simulink model "OmniServerSim_v2021b"  (R2021b)
settings: Solver=FixedStepAuto  StartTime=0.0  StopTime=inf  FixedStep=0.002  MaxStep=1e-2  RelTol=1e-3
model workspace (MATLAB code in the model file):
  | % function MacroDef()
  | 
  | % //Omni端数据的state定义
  | % #define OMNI_SEND_STATE_ERROR -100
  | global OMNI_SEND_STATE_ERROR
  | OMNI_SEND_STATE_ERROR = (-100);
  | % #define OMNI_SEND_STATE_EMPTY 0
  | global OMNI_SEND_STATE_EMPTY
  | OMNI_SEND_STATE_EMPTY = (0);
  | % #define OMNI_SEND_STATE_HEARTBEAT 10
  | global OMNI_SEND_STATE_HEARTBEAT
  | OMNI_SEND_STATE_HEARTBEAT = (10);
  | % #define OMNI_SEND_STATE_SYN 20
  | global OMNI_SEND_STATE_SYN
  | OMNI_SEND_STATE_SYN = (20);
  | % #define OMNI_SEND_STATE_ONLY_NOTE 30
  | global OMNI_SEND_STATE_ONLY_NOTE
  | OMNI_SEND_STATE_ONLY_NOTE = (30);
  | % #define OMNI_SEND_STATE_CURRENT_CORE 100
  | global OMNI_SEND_STATE_CURRENT_CORE
  | OMNI_SEND_STATE_CURRENT_CORE = (100);
  | % #define OMNI_SEND_STATE_LAST_CORE 101
  | global OMNI_SEND_STATE_LAST_CORE
  | OMNI_SEND_STATE_LAST_CORE = (101);
  | % #define OMNI_SEND_STATE_CURRENT_POSE 200
  | global OMNI_SEND_STATE_CURRENT_POSE
  | OMNI_SEND_STATE_CURRENT_POSE = (200);
  | % #define OMNI_SEND_STATE_LAST_POSE 201
  | global OMNI_SEND_STATE_LAST_POSE
  | OMNI_SEND_STATE_LAST_POSE = (201);
  | % #define OMNI_SEND_STATE_CURRENT_FORCE 300
  | global OMNI_SEND_STATE_CURRENT_FORCE
  | OMNI_SEND_STATE_CURRENT_FORCE = (300);
  | % #define OMNI_SEND_STATE_LAST_FORCE 301
  | global OMNI_SEND_STATE_LAST_FORCE
  | OMNI_SEND_STATE_LAST_FORCE = (301);
  | % #define OMNI_RCV_STATE_EMPTY 1000
  | global OMNI_RCV_STATE_EMPTY
  | OMNI_RCV_STATE_EMPTY = (1000);
  | % #define OMNI_RCV_STATE_HEARTBEAT 1010
  | global OMNI_RCV_STATE_HEARTBEAT
  | OMNI_RCV_STATE_HEARTBEAT = (1010);
  | % #define OMNI_RCV_STATE_TRIGGER 1020
  | global OMNI_RCV_STATE_TRIGGER
  | OMNI_RCV_STATE_TRIGGER = (1020);
  | % #define OMNI_RCV_STATE_CONFIG 1100
  | global OMNI_RCV_STATE_CONFIG
  | OMNI_RCV_STATE_CONFIG = (1100);
  | % #define OMNI_RCV_STATE_FORCE 1300
  | global OMNI_RCV_STATE_FORCE
  | OMNI_RCV_STATE_FORCE = (1300);
  | % #define OMNI_RCV_STATE_TORQUE 1301
  | global OMNI_RCV_STATE_TORQUE
  | OMNI_RCV_STATE_TORQUE = (1301);
  | 
  | % end
libraries: slrealtimeiplib x3, sldrtlib x2, simulink x1
settings Model: Creator=WDDSC  LastModifiedBy=WDDSC
settings DebuggingCC: UnconnectedInputMsg=none  UnconnectedOutputMsg=none  UnconnectedLineMsg=none
settings ModelReferenceCC: EnableRefExpFcnMdlSchedulingChecks=off
settings RTWCC: DLArmComputeVersion=20.02.1

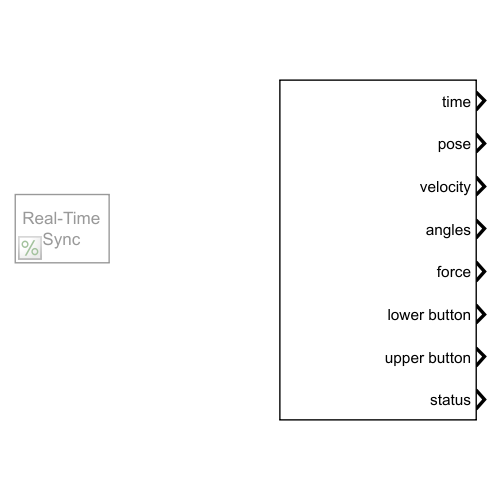
[thumbnail: Simulink's stored preview of the top-level diagram]
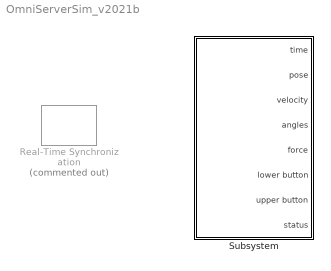
== system OmniServerSim_v2021b ==
  Real-Time Synchronization : sldrtlib/Real-Time Synchronization  Commented=on  SampleTime=0.002  MaxMissedTicks=inf  ShowMissedTicks=off  YieldWhenWaiting=off
  Subsystem : Subsystem  mask{Time=on}
      mask DialogControl ParameterGroupVar Prompt: 参数

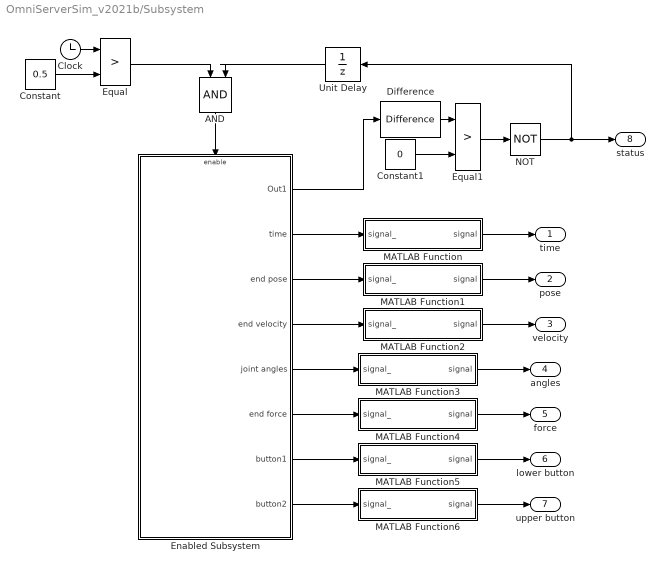
== system OmniServerSim_v2021b/Subsystem ==
  AND : Logic  IconShape=distinctive  AllPortsSameDT=off  OutDataTypeStr=boolean
  Clock : Clock
  Constant : Constant  Value=0.5
  Constant1 : Constant  Value=0
  Difference : simulink/Discrete/Difference  ICPrevInput=0.0  OutMin=[]  OutMax=[]  OutDataType=fixdt(1, 16)  OutScaling=2^-10  DoSatur=off
  Enabled Subsystem : Subsystem  TreatAsAtomicUnit=on
  Equal : RelationalOperator  Operator=>  OutDataTypeStr=boolean  RndMeth=Simplest
  Equal1 : RelationalOperator  Operator=>  OutDataTypeStr=boolean  RndMeth=Simplest
  MATLAB Function : MATLAB Function  TreatAsAtomicUnit=on  mask{Mode=Hold on (Keep the last value)}
      mask prompts: Mode "Choose the mode to substitute "nan""
      mask init:
      | Mode = get_param(gcb, "Mode");
      | disp(Mode);
  MATLAB Function1 : MATLAB Function  TreatAsAtomicUnit=on  mask{Mode=Hold on (Keep the last value)}
      mask prompts: Mode "Choose the mode to substitute "nan""
      mask init:
      | Mode = get_param(gcb, "Mode");
      | disp(Mode);
  MATLAB Function2 : MATLAB Function  TreatAsAtomicUnit=on  mask{Mode=Hold on (Keep the last value)}
      mask prompts: Mode "Choose the mode to substitute "nan""
      mask init:
      | Mode = get_param(gcb, "Mode");
      | disp(Mode);
  MATLAB Function3 : MATLAB Function  TreatAsAtomicUnit=on  mask{Mode=Hold on (Keep the last value)}
      mask prompts: Mode "Choose the mode to substitute "nan""
      mask init:
      | Mode = get_param(gcb, "Mode");
      | disp(Mode);
  MATLAB Function4 : MATLAB Function  TreatAsAtomicUnit=on  mask{Mode=Hold on (Keep the last value)}
      mask prompts: Mode "Choose the mode to substitute "nan""
      mask init:
      | Mode = get_param(gcb, "Mode");
      | disp(Mode);
  MATLAB Function5 : MATLAB Function  TreatAsAtomicUnit=on  mask{Mode=Hold on (Keep the last value)}
      mask prompts: Mode "Choose the mode to substitute "nan""
      mask init:
      | Mode = get_param(gcb, "Mode");
      | disp(Mode);
  MATLAB Function6 : MATLAB Function  TreatAsAtomicUnit=on  mask{Mode=Hold on (Keep the last value)}
      mask prompts: Mode "Choose the mode to substitute "nan""
      mask init:
      | Mode = get_param(gcb, "Mode");
      | disp(Mode);
  NOT : Logic  Operator=NOT  IconShape=distinctive  AllPortsSameDT=off  OutDataTypeStr=boolean
  Unit Delay : UnitDelay  SampleTime=-1  HasFrameUpgradeWarning=on
  time : Outport
  pose : Outport  Port=2
  velocity : Outport  Port=3
  angles : Outport  Port=4
  force : Outport  Port=5
  lower button : Outport  Port=6
  upper button : Outport  Port=7
  status : Outport  Port=8
  wires:
  NOT/1 -> status/1, Unit Delay/1
  AND/1 -> Enabled Subsystem/Enable
  Equal/1 -> AND/1
  Difference/1 -> Equal1/1
  Constant1/1 -> Equal1/2
  Enabled Subsystem/1(Out1) -> Difference/1
  Clock/1 -> Equal/1
  Constant/1 -> Equal/2
  Equal1/1 -> NOT/1
  Unit Delay/1 -> AND/2
  Enabled Subsystem/2(time) -> MATLAB Function/1(signal_)
  MATLAB Function/1(signal) -> time/1
  MATLAB Function1/1(signal) -> pose/1
  Enabled Subsystem/3(end pose) -> MATLAB Function1/1(signal_)
  MATLAB Function2/1(signal) -> velocity/1
  Enabled Subsystem/4(end velocity) -> MATLAB Function2/1(signal_)
  MATLAB Function3/1(signal) -> angles/1
  Enabled Subsystem/5(joint angles) -> MATLAB Function3/1(signal_)
  MATLAB Function4/1(signal) -> force/1
  Enabled Subsystem/6(end force) -> MATLAB Function4/1(signal_)
  MATLAB Function5/1(signal) -> lower button/1
  Enabled Subsystem/7(button1) -> MATLAB Function5/1(signal_)
  MATLAB Function6/1(signal) -> upper button/1
  Enabled Subsystem/8(button2) -> MATLAB Function6/1(signal_)

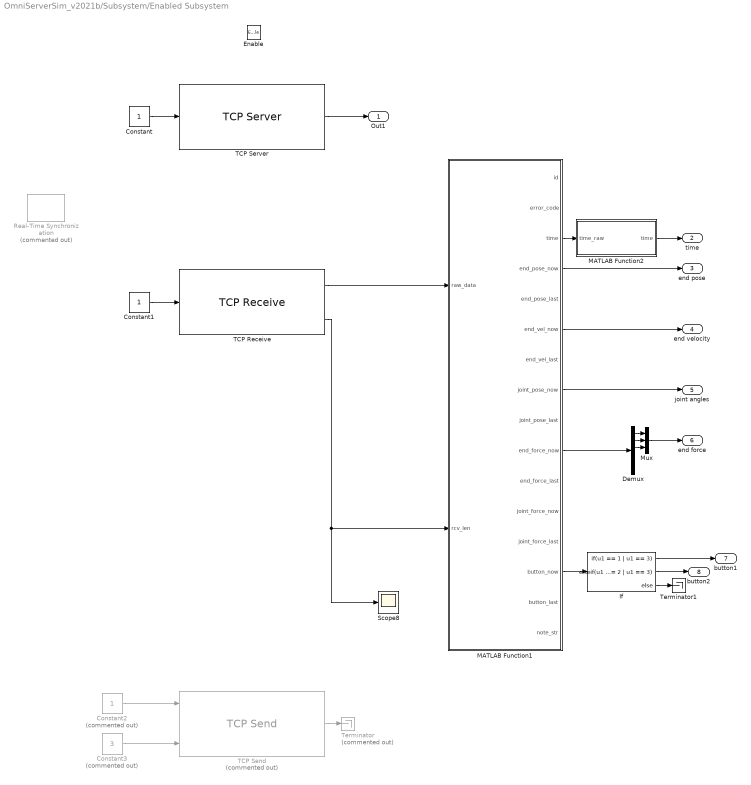
== system OmniServerSim_v2021b/Subsystem/Enabled Subsystem ==
  Enable : EnablePort  StatesWhenEnabling=reset
  Constant : Constant
  Constant1 : Constant
  Constant2 : Constant  Commented=on
  Constant3 : Constant  Commented=on  Value=3
  Demux : Demux  Outputs=6
  If : If  IfExpression=u1 == 1 | u1 == 3  ElseIfExpressions=u1 == 2 | u1 == 3
  MATLAB Function1 : MATLAB Function  TreatAsAtomicUnit=on
  MATLAB Function2 : MATLAB Function  TreatAsAtomicUnit=on
  Mux : Mux  Inputs=3
  Real-Time Synchronization : sldrtlib/Real-Time Synchronization  Commented=on  SampleTime=1e-2  MaxMissedTicks=inf  ShowMissedTicks=off  YieldWhenWaiting=off
  Scope8 : Scope
  TCP Receive : slrealtimeiplib/TCP Receive  socketAddPortVal=Server: 127.0.0.1:10301  rcvWidth=40960  sampleTime=-1
  TCP Send : slrealtimeiplib/TCP Send  Commented=on  socketAddPortVal=Server: 127.0.0.1:10301  sampleTime=-1
  TCP Server : slrealtimeiplib/TCP Server  Priority=-1  useHostTargetConn=off  serverAddress=127.0.0.1  serverPort=10301
  Terminator : Terminator  Commented=on
  Terminator1 : Terminator
  Out1 : Outport
  time : Outport  Port=2
  end pose : Outport  Port=3
  end velocity : Outport  Port=4
  joint angles : Outport  Port=5
  end force : Outport  Port=6
  button1 : Outport  Port=7
  button2 : Outport  Port=8
  wires:
  TCP Server/1 -> Out1/1
  Constant/1 -> TCP Server/1
  TCP Receive/1 -> MATLAB Function1/1(raw_data)
  Constant1/1 -> TCP Receive/1
  TCP Receive/2 -> Scope8/1, MATLAB Function1/2(rcv_len)
  MATLAB Function1/3(time) -> MATLAB Function2/1(time_raw)
  Constant2/1 -> TCP Send/1
  Constant3/1 -> TCP Send/3
  TCP Send/1 -> Terminator/1
  MATLAB Function2/1(time) -> time/1
  MATLAB Function1/4(end_pose_now) -> end pose/1
  MATLAB Function1/6(end_vel_now) -> end velocity/1
  MATLAB Function1/8(joint_pose_now) -> joint angles/1
  MATLAB Function1/10(end_force_now) -> Demux/1
  MATLAB Function1/14(button_now) -> If/1
  If/1 -> button1/1
  If/2 -> button2/1
  If/3 -> Terminator1/1
  Demux/1 -> Mux/1
  Demux/2 -> Mux/2
  Demux/3 -> Mux/3
  Mux/1 -> end force/1

== matlab function OmniServerSim_v2021b/Subsystem/MATLAB Function4 ==
  data: signal_ input; signal output; Mode parameter
function signal = killNan(signal_, Mode)

persistent signal_last;

if isempty(signal_last)
    signal_last = nan(size(signal_));
end
signal = nan(size(signal_));

switch Mode
    case 1 %保持上一时刻值
        for i=1:length(signal_)
            if isnan(signal_(i))
                if isnan(signal_last)
                    signal(i) = nan;
                else
                    signal(i) = signal_last(i);
                end
            else
                signal(i) = signal_(i);
            end
        end
    case 2 %置0
        for i=1:length(signal_)
            if isnan(signal_(i))
                signal(i) = 0.0;
            else
                signal(i) = signal_(i);
            end
        end
    case 3 %保持nan
        signal = signal_;
end

signal_last = signal;

== matlab function OmniServerSim_v2021b/Subsystem/MATLAB Function5 ==
  data: signal_ input; signal output; Mode parameter
function signal = killNan(signal_, Mode)

persistent signal_last;

if isempty(signal_last)
    signal_last = nan(size(signal_));
end
signal = nan(size(signal_));

switch Mode
    case 1 %保持上一时刻值
        for i=1:length(signal_)
            if isnan(signal_(i))
                if isnan(signal_last)
                    signal(i) = nan;
                else
                    signal(i) = signal_last(i);
                end
            else
                signal(i) = signal_(i);
            end
        end
    case 2 %置0
        for i=1:length(signal_)
            if isnan(signal_(i))
                signal(i) = 0.0;
            else
                signal(i) = signal_(i);
            end
        end
    case 3 %保持nan
        signal = signal_;
end

signal_last = signal;

== matlab function OmniServerSim_v2021b/Subsystem/MATLAB Function6 ==
  data: signal_ input; signal output; Mode parameter
function signal = killNan(signal_, Mode)

persistent signal_last;

if isempty(signal_last)
    signal_last = nan(size(signal_));
end
signal = nan(size(signal_));

switch Mode
    case 1 %保持上一时刻值
        for i=1:length(signal_)
            if isnan(signal_(i))
                if isnan(signal_last)
                    signal(i) = nan;
                else
                    signal(i) = signal_last(i);
                end
            else
                signal(i) = signal_(i);
            end
        end
    case 2 %置0
        for i=1:length(signal_)
            if isnan(signal_(i))
                signal(i) = 0.0;
            else
                signal(i) = signal_(i);
            end
        end
    case 3 %保持nan
        signal = signal_;
end

signal_last = signal;

== matlab function OmniServerSim_v2021b/Subsystem/Enabled Subsystem/MATLAB Function1 ==
  data: id output double size=1; error_code output size=1; time output size=1; end_pose_now output; end_pose_last output; end_vel_now output; end_vel_last output; joint_pose_now output; joint_pose_last output; end_force_now output; end_force_last output; joint_force_now output; joint_force_last output; button_now output; button_last output; note_str output; raw_data input; rcv_len input
% function [trunc_data, id, state, error_code, time] = GrabMsg(raw_data, rcv_len)
% function [error_code, ...
%     end_position, button] = GrabMsg(raw_data, rcv_len)
function [id, error_code, time, ...
    end_pose_now, end_pose_last, ...
    end_vel_now, end_vel_last, ...
    joint_pose_now, joint_pose_last, ...
    end_force_now, end_force_last, ...
    joint_force_now, joint_force_last, ...
    button_now, button_last, ...
    note_str] = GrabMsg(raw_data, rcv_len)

%% 读空数据后，截取一帧

%初始化输出
id = -1;
%state = nan;
error_code = nan;
time = -1;
[end_pose_now, end_pose_last, ...
end_vel_now, end_vel_last, ...
joint_pose_now, joint_pose_last, ...
end_force_now, end_force_last, ...
joint_force_now, joint_force_last] = deal(nan(6,1));
[button_now, button_last] = deal(nan);
note_str = "";

omni_status = getEmptyStatus();

%若接受的数据长度正常（256的倍数），开始处理
if rcv_len <= 0
    error_code = -1;
elseif mod(rcv_len,256) ~= 0
    error_code = -2;
else
    error_code = 0; %只有err=0才代表接受数据成功
    % 遍历所有数据帧，尽量不漏消息
    for iframe = 1 : rcv_len/256
        trunc_data = raw_data((iframe-1)*256+1 : iframe*256);
        tmp = double(typecast(uint8(trunc_data(5:8)), 'int32'));
        id = max([id, tmp(1)]);
        %state = double(typecast(uint8(trunc_data(9:12)), 'int32'));
        tmp = max(double(typecast(uint8(trunc_data(13:16)), 'int32')));
        error_code = max([error_code, tmp(1)]);
        tmp = double(typecast(uint8(trunc_data(17:24)), 'int64'));
        time = max([time, tmp(1)]);
        omni_status = solveStatus(trunc_data, omni_status);
    end
end

%输出量赋值

end_pose_now(1:3) = omni_status.end_position_now(1:3);
end_pose_now(4:6) = omni_status.joint_angles_now(1:3);
end_pose_last(1:3) = omni_status.end_position_last(1:3);
end_pose_last(4:6) = omni_status.joint_angles_last(1:3);

end_vel_now(1:3) = omni_status.end_velocity_now(1:3);
end_vel_now(4:6) = omni_status.gimbal_velocity_now(1:3);
end_vel_last(1:3) = omni_status.end_velocity_last(1:3);
end_vel_last(4:6) = omni_status.gimbal_velocity_last(1:3);

joint_pose_now(1:3) = omni_status.joint_angles_now(1:3);
joint_pose_now(4:6) = omni_status.gimbal_angles_now(1:3);
joint_pose_last(1:3) = omni_status.joint_angles_last(1:3);
joint_pose_last(4:6) = omni_status.gimbal_angles_last(1:3);

end_force_now(1:3) = omni_status.end_force_now(1:3);
end_force_now(4:6) = omni_status.end_torque_now(1:3);
end_force_last(1:3) = omni_status.end_force_last(1:3);
end_force_last(4:6) = omni_status.end_torque_last(1:3);

joint_force_now(1:3) = omni_status.joint_torque_now(1:3);
joint_force_now(4:6) = omni_status.gimbal_torque_now(1:3);
joint_force_last(1:3) = omni_status.joint_torque_last(1:3);
joint_force_last(4:6) = omni_status.gimbal_torque_last(1:3);

button_now = omni_status.button_now(1);
button_last = omni_status.button_last(1);

note_str = omni_status.note_str;

== matlab function OmniServerSim_v2021b/Subsystem/MATLAB Function ==
  data: signal_ input; signal output; Mode parameter
function signal = killNan(signal_, Mode)

persistent signal_last;

if isempty(signal_last)
    signal_last = nan(size(signal_));
end
signal = nan(size(signal_));

switch Mode
    case 1 %保持上一时刻值
        for i=1:length(signal_)
            if isnan(signal_(i))
                if isnan(signal_last)
                    signal(i) = nan;
                else
                    signal(i) = signal_last(i);
                end
            else
                signal(i) = signal_(i);
            end
        end
    case 2 %置0
        for i=1:length(signal_)
            if isnan(signal_(i))
                signal(i) = 0.0;
            else
                signal(i) = signal_(i);
            end
        end
    case 3 %保持nan
        signal = signal_;
end

signal_last = signal;

== matlab function OmniServerSim_v2021b/Subsystem/Enabled Subsystem/MATLAB Function2 ==
  data: time_raw input; time output
function time  = solveTime(time_raw)

persistent time_first;
if isempty(time_first)
    time_first = nan;
end
if ~isnan(time_raw) && time_raw > 0
    if isnan(time_first)
        time_first = time_raw;
    end
    time = 1e-6*(time_raw - time_first);
else
    time = nan;
end

== matlab function OmniServerSim_v2021b/Subsystem/MATLAB Function1 ==
  data: signal_ input; signal output; Mode parameter
function signal = killNan(signal_, Mode)

persistent signal_last;

if isempty(signal_last)
    signal_last = nan(size(signal_));
end
signal = nan(size(signal_));

switch Mode
    case 1 %保持上一时刻值
        for i=1:length(signal_)
            if isnan(signal_(i))
                if isnan(signal_last)
                    signal(i) = nan;
                else
                    signal(i) = signal_last(i);
                end
            else
                signal(i) = signal_(i);
            end
        end
    case 2 %置0
        for i=1:length(signal_)
            if isnan(signal_(i))
                signal(i) = 0.0;
            else
                signal(i) = signal_(i);
            end
        end
    case 3 %保持nan
        signal = signal_;
end

signal_last = signal;

== matlab function OmniServerSim_v2021b/Subsystem/MATLAB Function2 ==
  data: signal_ input; signal output; Mode parameter
function signal = killNan(signal_, Mode)

persistent signal_last;

if isempty(signal_last)
    signal_last = nan(size(signal_));
end
signal = nan(size(signal_));

switch Mode
    case 1 %保持上一时刻值
        for i=1:length(signal_)
            if isnan(signal_(i))
                if isnan(signal_last)
                    signal(i) = nan;
                else
                    signal(i) = signal_last(i);
                end
            else
                signal(i) = signal_(i);
            end
        end
    case 2 %置0
        for i=1:length(signal_)
            if isnan(signal_(i))
                signal(i) = 0.0;
            else
                signal(i) = signal_(i);
            end
        end
    case 3 %保持nan
        signal = signal_;
end

signal_last = signal;

== matlab function OmniServerSim_v2021b/Subsystem/MATLAB Function3 ==
  data: signal_ input; signal output; Mode parameter
function signal = killNan(signal_, Mode)

persistent signal_last;

if isempty(signal_last)
    signal_last = nan(size(signal_));
end
signal = nan(size(signal_));

switch Mode
    case 1 %保持上一时刻值
        for i=1:length(signal_)
            if isnan(signal_(i))
                if isnan(signal_last)
                    signal(i) = nan;
                else
                    signal(i) = signal_last(i);
                end
            else
                signal(i) = signal_(i);
            end
        end
    case 2 %置0
        for i=1:length(signal_)
            if isnan(signal_(i))
                signal(i) = 0.0;
            else
                signal(i) = signal_(i);
            end
        end
    case 3 %保持nan
        signal = signal_;
end

signal_last = signal;
